simulink model "simulador2017bVALIDATION_v2"  (R2017b)
settings: Solver=FixedStepAuto  StartTime=0.0  StopTime=60*3  FixedStep=0.001  MaxStep=0.001  RelTol=1e-3
values from neighbouring files (symbols this model uses):
  b = 2.9    [FUN_v2.m]    (also in ratesDerivatives.m = (1/windowSize)*ones(1,windowSize))
  c_bar = 0.19    [FUN_v2.m]
  CD_deltae = x(5)    [FUN_v2.m]
  CDp = x(1)    [FUN_v2.m]
  CDq = x(4)    [FUN_v2.m]
  CL0 = x(6)    [FUN_v2.m]
  CL_alpha = x(7)    [FUN_v2.m]
  Cl_beta = x(15)    [FUN_v2.m]
  Cl_da = x(19)    [FUN_v2.m]
  CL_deltae = x(9)    [FUN_v2.m]
  Cl_dr = x(18)    [FUN_v2.m]
  Cl_p = x(16)    [FUN_v2.m]
  Cl_r = x(17)    [FUN_v2.m]
  CLq = x(8)    [FUN_v2.m]
  Cm0 = x(20)    [FUN_v2.m]
  Cm_alpha = x(21)    [FUN_v2.m]
  Cm_de = x(23)    [FUN_v2.m]
  Cm_q = x(22)    [FUN_v2.m]
  Cn_beta = x(24)    [FUN_v2.m]
  Cn_da = x(28)    [FUN_v2.m]
  Cn_dr = x(27)    [FUN_v2.m]
  Cn_p = x(25)    [FUN_v2.m]
  Cn_r = x(26)    [FUN_v2.m]
  Cy_beta = x(10)    [FUN_v2.m]
  Cy_da = x(13)    [FUN_v2.m]
  Cy_dr = x(14)    [FUN_v2.m]
  Cy_p = x(11)    [FUN_v2.m]
  Cy_r = x(12)    [FUN_v2.m]
  deltat_pts = parameters.deltat_pts    [propulsiveModel.m]
  k1 = x(3)    [FUN_v2.m]
  k2 = x(2)    [FUN_v2.m]
  M = parameters.M    [propulsiveModel.m]
  mass = 11    [FUN_v2.m]
  q = XDATA(:,5)    [FUN_v2.m]    (also in NONLINEAR_IDENTIFICATION_v2.m = myResize(q_meas); ratesDerivatives.m = q_meas)
  r = XDATA(:,6)    [FUN_v2.m]    (also in NONLINEAR_IDENTIFICATION_v2.m = myResize(r_meas); ratesDerivatives.m = r_meas)
  RPM_pts = parameters.RPM_pts    [propulsiveModel.m]
  T = table(xfit,xreal,relErrorPorcentage','RowNames',coeffName)    [NONLINEAR_IDENTIFICATION_v2.m]    (also in propulsiveModel.m = parameters.T)
  V = sqrt(u.*u+v.*v+w.*w)    [NoisySignals_plot.m]
undefined symbols (not defined in the file or in its folder): Cl0, Cm_df, Cn0, Cx_df, Cx_dr, Cy0, Cz_df, delta_max, Earth, F, Light, maxRPM, MIL, N, Vw_unif, WGS84
libraries: aerolibwind2 x3, aerolibtransform2 x2, aerolibasang x2, aerolibfltsims x1, simulink_extras x1, aerolibatmos2 x1, shared6dof x1, aerolibadyn x1
(part 2 of 2)

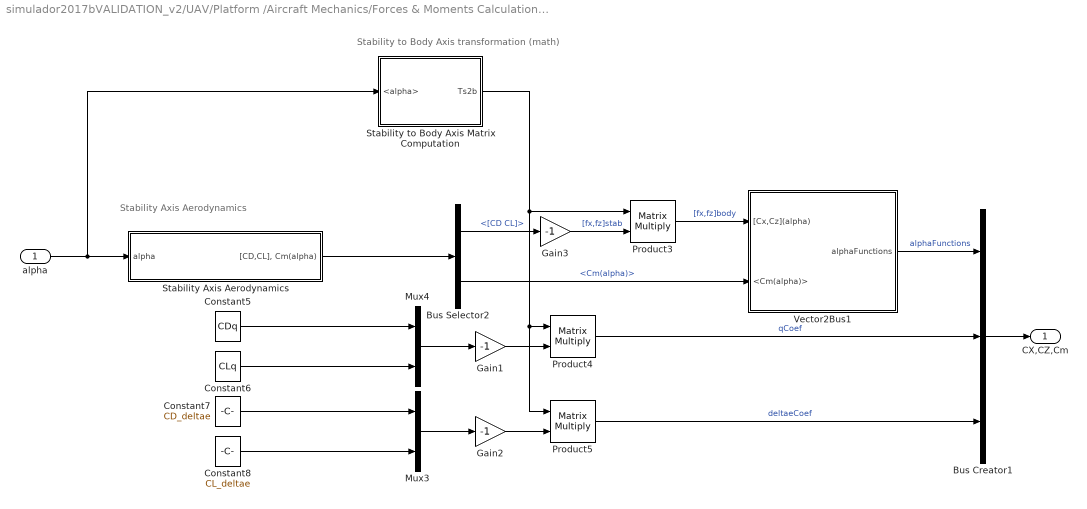
== system simulador2017bVALIDATION_v2/UAV/Platform /Aircraft Mechanics/Forces & Moments Calculation/Aerodynamic Coefficients /Longitudinal Aerodynamics (Cx, Cz, Cm coefficients) ==
  note: Stability Axis Aerodynamics
  note: Stability to Body Axis transformation (math)
  "alpha " : Inport
  Bus Creator1 : BusCreator  Inputs=3
  Bus Selector2 : BusSelector  OutputSignals=[CD CL],Cm(alpha)
  Constant5 : Constant  Value=CDq
      mask Display: port_label('output',1,'C_{D_q}','texmode','on')
  Constant6 : Constant  Value=CLq
      mask Display: port_label('output',1,'C_{L_q}','texmode','on')
  Constant7 : Constant  Value=CD_deltae
      mask Display: port_label('output',1,'C_{D_{\delta_e}}','texmode','on')
  Constant8 : Constant  Value=CL_deltae
      mask Display: port_label('output',1,'C_{L_{\delta_e}}','texmode','on')
  Gain1 : Gain  Gain=-1
  Gain2 : Gain  Gain=-1
  Gain3 : Gain  Gain=-1
  Mux3 : Mux  Inputs=2
  Mux4 : Mux  Inputs=2
  Product3 : Product  Multiplication=Matrix(*)
  Product4 : Product  Multiplication=Matrix(*)
  Product5 : Product  Multiplication=Matrix(*)
  Stability Axis Aerodynamics : Subsystem
      mask Display:
      | port_label('input',1,'\alpha','texmode','on')
      | port_label('output',1,'[C_D(\alpha),C_L(\alpha)], C_m(\alpha)','texmode','on')
  Stability to Body Axis Matrix Computation : Subsystem
      mask Display:
      | port_label('input',1,'\alpha','texmode','on')
      | port_label('output',1,'T_{s2b}(\alpha)','texmode','on')
  Vector2Bus1 : Subsystem
      mask Display:
      | port_label('input',1,'[C_X(\alpha), C_Z(\alpha)]','texmode','on')
      | port_label('input',2,'C_m(\alpha)','texmode','on')
      | port_label('output',1,'C_X(\alpha),C_Z(\alpha),C_m(\alpha)','texmode','on')
  CX,CZ,Cm : Outport
  wires:
  Bus Creator1/1 -> CX,CZ,Cm/1
  Gain3/1 -> Product3/2  "[fx,fz]stab"
  Stability Axis Aerodynamics/1("[CD,CL], Cm(alpha)") -> Bus Selector2/1
  Constant7/1 -> Mux3/1
  Stability to Body Axis Matrix Computation/1(Ts2b) -> Product5/1, Product4/1, Product3/1
  Product4/1 -> Bus Creator1/2  "qCoef"
  Bus Selector2/1 -> Gain3/1  "<[CD CL]>"
  Product5/1 -> Bus Creator1/3  "deltaeCoef"
  Product3/1 -> Vector2Bus1/1("[Cx,Cz](alpha)")  "[fx,fz]body"
  Bus Selector2/2 -> Vector2Bus1/2(<Cm(alpha)>)  "<Cm(alpha)>"
  Constant8/1 -> Mux3/2
  Vector2Bus1/1(alphaFunctions) -> Bus Creator1/1  "alphaFunctions"
  Constant6/1 -> Mux4/2
  Constant5/1 -> Mux4/1
  Mux3/1 -> Gain2/1
  Gain2/1 -> Product5/2
  Mux4/1 -> Gain1/1
  Gain1/1 -> Product4/2
  "alpha "/1 -> Stability Axis Aerodynamics/1(alpha), Stability to Body Axis Matrix Computation/1(<alpha>)

== system simulador2017bVALIDATION_v2/UAV/Platform /Aircraft Mechanics/Forces & Moments Calculation/Aerodynamic Coefficients /alpha-beta Coefficients ==
  beta : Inport  Unit=radian
  Bus Element In : Inport  Port=2  PortName=Longitudinal Aerodynamics  Element=Cm(alpha)
  Bus Element In1 : Inport  Port=2  PortName=Longitudinal Aerodynamics  Element=Cz(alpha)
  Bus Element In2 : Inport  Port=2  PortName=Longitudinal Aerodynamics  Element=Cx(alpha)
  Gain1 : Gain  Gain=Cn_beta  SaturateOnIntegerOverflow=on  OutDataTypeStr=Inherit: Same as input  ParamDataTypeStr=Inherit: Same as input
  Gain3 : Gain  Gain=Cy_beta  SaturateOnIntegerOverflow=on  OutDataTypeStr=Inherit: Same as input  ParamDataTypeStr=Inherit: Same as input
  Gain6 : Gain  Gain=Cl_beta  SaturateOnIntegerOverflow=on  OutDataTypeStr=Inherit: Same as input  ParamDataTypeStr=Inherit: Same as input
  Lateral Dynamics Constants : Constant  Value=[0,Cy0,0,Cl0,0,Cn0]
  Mux1 : Mux  Inputs=6
  Sum4 : Sum  Inputs=|++  SaturateOnIntegerOverflow=on
  Coefficients : Outport
  wires:
  Lateral Dynamics Constants/1 -> Sum4/2
  Sum4/1 -> Coefficients/1
  Mux1/1 -> Sum4/1
  Gain3/1 -> Mux1/2  "Cy"
  Gain6/1 -> Mux1/4  "Cl"
  beta/1 -> Gain1/1, Gain6/1, Gain3/1  "beta"
  Gain1/1 -> Mux1/6
  Bus Element In/1 -> Mux1/5
  Bus Element In1/1 -> Mux1/3
  Bus Element In2/1 -> Mux1/1

== system simulador2017bVALIDATION_v2/UAV/Platform /Aircraft Mechanics/Forces & Moments Calculation/Propulsion/1 dim to 6 dim1 ==
  Tprop : Inport
  Qprop : Inport  Port=2
  Bus Creator : BusCreator  Inputs=2
  Constant : Constant  Value=0
  Mux : Mux  Inputs=3
  Mux1 : Mux  Inputs=3
  Propulsion BUS : Outport
  wires:
  Bus Creator/1 -> Propulsion BUS/1
  Constant/1 -> Mux/3, Mux/2, Mux1/2, Mux1/3
  Qprop/1 -> Mux1/1
  Tprop/1 -> Mux/1
  Mux/1 -> Bus Creator/1  "Tprop"
  Mux1/1 -> Bus Creator/2  "Mprop"

== system simulador2017bVALIDATION_v2/UAV/Platform /Aircraft Mechanics/Forces & Moments Calculation/Propulsion/Propeller ==
  RPM : Inport
  u : Inport  Port=2
  1-D Lookup Table : Lookup_n-D  BreakpointsForDimension1=N  BreakpointsForDimension2=V  Table=T  InternalRulePriority=Speed  RndMeth=Simplest  InputSameDT=on
  1-D Lookup Table1 : Lookup_n-D  BreakpointsForDimension1=N  BreakpointsForDimension2=V  Table=M  InternalRulePriority=Speed  RndMeth=Simplest  InputSameDT=on
  Tables work with RPM/1000 : Gain  Gain=1/1000
  Tprop : Outport
  Qprop : Outport  Port=2
  wires:
  1-D Lookup Table/1 -> Tprop/1
  u/1 -> 1-D Lookup Table/2, 1-D Lookup Table1/2
  1-D Lookup Table1/1 -> Qprop/1
  RPM/1 -> Tables work with RPM/1000/1
  Tables work with RPM/1000/1 -> 1-D Lookup Table1/1, 1-D Lookup Table/1

== system simulador2017bVALIDATION_v2/UAV/Platform /Aircraft Mechanics/Forces & Moments Calculation/Aerodynamic Coefficients /Actuator Increments/Aileron ==
  note: Se ha despreciado el efecto del angulo de ataque,
      | que afecta a las superficies de control si es muy alto
  deltaa : Inport  Unit=rad
  Gain1 : Gain  Gain=0  SaturateOnIntegerOverflow=on  OutDataTypeStr=Inherit: Same as input  ParamDataTypeStr=Inherit: Same as input
  Gain2 : Gain  Gain=Cy_da  SaturateOnIntegerOverflow=on  OutDataTypeStr=Inherit: Same as input  ParamDataTypeStr=Inherit: Same as input
  Gain3 : Gain  Gain=0  SaturateOnIntegerOverflow=on  OutDataTypeStr=Inherit: Same as input  ParamDataTypeStr=Inherit: Same as input
  Gain4 : Gain  Gain=Cn_da  SaturateOnIntegerOverflow=on  OutDataTypeStr=Inherit: Same as input  ParamDataTypeStr=Inherit: Same as input
  Gain5 : Gain  Gain=0  SaturateOnIntegerOverflow=on  OutDataTypeStr=Inherit: Same as input  ParamDataTypeStr=Inherit: Same as input
  Gain6 : Gain  Gain=Cl_da  SaturateOnIntegerOverflow=on  OutDataTypeStr=Inherit: Same as input  ParamDataTypeStr=Inherit: Same as input
  Mux1 : Mux  Inputs=6
  delCoeff : Outport
  wires:
  Gain6/1 -> Mux1/4
  Gain1/1 -> Mux1/1  "Cx"
  Mux1/1 -> delCoeff/1
  Gain2/1 -> Mux1/2  "Cy"
  Gain3/1 -> Mux1/3  "Cz"
  Gain5/1 -> Mux1/5  "Cm"
  Gain4/1 -> Mux1/6
  deltaa/1 -> Gain2/1, Gain3/1, Gain5/1, Gain4/1, Gain6/1, Gain1/1

== system simulador2017bVALIDATION_v2/UAV/Platform /Aircraft Mechanics/Forces & Moments Calculation/Aerodynamic Coefficients /Actuator Increments/Elevator ==
  "Cx_deltae, Cz_deltae" : Inport
  deltae : Inport  Port=2
  Constant1 : Constant  Value=0
  Demux : Demux  Outputs=2
  Gain3 : Gain  Gain=Cm_de  SaturateOnIntegerOverflow=on  OutDataTypeStr=Inherit: Same as input  ParamDataTypeStr=Inherit: Same as input
  Mux1 : Mux  Inputs=6
  Product : Product
  Product1 : Product
  delCoeff : Outport
  wires:
  Gain3/1 -> Mux1/5
  Product1/1 -> Mux1/3
  Mux1/1 -> delCoeff/1
  Constant1/1 -> Mux1/4, Mux1/6, Mux1/2
  Product/1 -> Mux1/1
  "Cx_deltae, Cz_deltae"/1 -> Demux/1
  Demux/1 -> Product/1  "Cx_deltae"
  Demux/2 -> Product1/1  "Cz_deltae"
  deltae/1 -> Product/2, Product1/2, Gain3/1

== system simulador2017bVALIDATION_v2/UAV/Platform /Aircraft Mechanics/Forces & Moments Calculation/Aerodynamic Coefficients /Actuator Increments/Flap ==
  deltaf : Inport  Unit=rad
  Constant1 : Constant  Value=0
  Gain1 : Gain  Gain=Cx_df  SaturateOnIntegerOverflow=on  OutDataTypeStr=Inherit: Same as input  ParamDataTypeStr=Inherit: Same as input
  Gain3 : Gain  Gain=Cz_df  SaturateOnIntegerOverflow=on  OutDataTypeStr=Inherit: Same as input  ParamDataTypeStr=Inherit: Same as input
  Gain5 : Gain  Gain=Cm_df  SaturateOnIntegerOverflow=on  OutDataTypeStr=Inherit: Same as input  ParamDataTypeStr=Inherit: Same as input
  Mux1 : Mux  Inputs=6
  delCoeff : Outport
  wires:
  deltaf/1 -> Gain1/1, Gain3/1, Gain5/1  "df"
  Gain5/1 -> Mux1/5
  Mux1/1 -> delCoeff/1
  Constant1/1 -> Mux1/4, Mux1/6, Mux1/2
  Gain1/1 -> Mux1/1
  Gain3/1 -> Mux1/3

== system simulador2017bVALIDATION_v2/UAV/Platform /Aircraft Mechanics/Forces & Moments Calculation/Aerodynamic Coefficients /Actuator Increments/Rudder ==
  note: Se añade la contribucion en
      | resistencia del Rudder direccion X
  note: Se ha despreciado el efecto del angulo de ataque,
      | que afecta a las superficies de control si es muy alto
  deltar : Inport  Unit=rad
  Constant1 : Constant  Value=0
  Gain1 : Gain  Gain=Cl_dr  SaturateOnIntegerOverflow=on  OutDataTypeStr=Inherit: Same as input  ParamDataTypeStr=Inherit: Same as input
  Gain2 : Gain  Gain=Cn_dr  SaturateOnIntegerOverflow=on  OutDataTypeStr=Inherit: Same as input  ParamDataTypeStr=Inherit: Same as input
  Gain4 : Gain  Gain=Cy_dr  SaturateOnIntegerOverflow=on  OutDataTypeStr=Inherit: Same as input  ParamDataTypeStr=Inherit: Same as input
  Gain5 : Gain  Commented=on  Gain=Cx_dr  SaturateOnIntegerOverflow=on  OutDataTypeStr=Inherit: Same as input  ParamDataTypeStr=Inherit: Same as input
  Mux1 : Mux  Inputs=6
  delCoeff : Outport
  wires:
  Gain1/1 -> Mux1/4
  Gain2/1 -> Mux1/6
  Mux1/1 -> delCoeff/1
  Gain4/1 -> Mux1/2
  Constant1/1 -> Mux1/1, Mux1/5, Mux1/3
  deltar/1 -> Gain5/1, Gain4/1, Gain1/1, Gain2/1  "dr"

== system simulador2017bVALIDATION_v2/UAV/Platform /Aircraft Mechanics/Forces & Moments Calculation/Aerodynamic Coefficients /Body Rate Damping/p Coefficients ==
  Constant1 : Constant  Value=0
  Constant2 : Constant  Value=Cy_p
  Constant3 : Constant  Value=Cl_p
  Constant4 : Constant  Value=Cn_p
  Mux1 : Mux  Inputs=6
  p Coeff : Outport
  wires:
  Constant2/1 -> Mux1/2
  Mux1/1 -> p Coeff/1
  Constant1/1 -> Mux1/5, Mux1/3, Mux1/1
  Constant4/1 -> Mux1/6
  Constant3/1 -> Mux1/4

== system simulador2017bVALIDATION_v2/UAV/Platform /Aircraft Mechanics/Forces & Moments Calculation/Aerodynamic Coefficients /Body Rate Damping/q Coefficients ==
  qCoef : Inport
  Constant1 : Constant  Value=0
  Constant4 : Constant  Value=Cm_q
  Demux : Demux  Outputs=2
  Mux1 : Mux  Inputs=6
  delCoeff : Outport
  wires:
  Constant1/1 -> Mux1/6, Mux1/4, Mux1/2
  Constant4/1 -> Mux1/5
  Mux1/1 -> delCoeff/1
  qCoef/1 -> Demux/1
  Demux/1 -> Mux1/1  "Cx_q"
  Demux/2 -> Mux1/3  "Cz_q"

== system simulador2017bVALIDATION_v2/UAV/Platform /Aircraft Mechanics/Forces & Moments Calculation/Aerodynamic Coefficients /Body Rate Damping/r Coefficients ==
  Constant : Constant  Value=0
  Constant1 : Constant  Value=Cy_r
  Constant2 : Constant  Value=Cl_r
  Constant4 : Constant  Value=Cn_r
  Mux1 : Mux  Inputs=6
  r Coeff : Outport
  wires:
  Constant/1 -> Mux1/5, Mux1/3, Mux1/1
  Constant1/1 -> Mux1/2
  Constant4/1 -> Mux1/6
  Constant2/1 -> Mux1/4
  Mux1/1 -> r Coeff/1

== system simulador2017bVALIDATION_v2/UAV/Platform /Aircraft Mechanics/Forces & Moments Calculation/Aerodynamic Coefficients /Longitudinal Aerodynamics (Cx, Cz, Cm coefficients)/Stability Axis Aerodynamics ==
  note: CD
  alpha : Inport
  Constant1 : Constant  Value=CL0
  Constant2 : Constant  Value=Cm0
  Constant3 : Constant  Value=CDp
  Gain1 : Gain  Gain=k1
  Gain2 : Gain  Gain=k2
  Gain4 : Gain  Gain=CL_alpha
  Gain5 : Gain  Gain=Cm_alpha
  Math Function : Math  Operator=square  SaturateOnIntegerOverflow=on
  Mux : Mux  Inputs=3
  Sum : Sum  Inputs=|++
  Sum1 : Sum  Inputs=|++
  Sum2 : Sum  Inputs=+++
  Vector2Bus : Subsystem
  "[CD,CL], Cm(alpha)" : Outport
  wires:
  Gain4/1 -> Sum/1
  Gain5/1 -> Sum1/1
  Vector2Bus/1("[CD,CL], Cm") -> "[CD,CL], Cm(alpha)"/1
  Constant1/1 -> Sum/2
  Constant2/1 -> Sum1/2
  Sum1/1 -> Mux/3  "Cm"
  Mux/1 -> Vector2Bus/1("[CD,CL,Cm]")
  Sum2/1 -> Mux/1  "CD"
  Sum/1 -> Gain2/1, Math Function/1, Mux/2  "CL"
  Constant3/1 -> Sum2/3
  alpha/1 -> Gain5/1, Gain4/1
  Gain2/1 -> Sum2/2
  Math Function/1 -> Gain1/1  "CL2"
  Gain1/1 -> Sum2/1

== system simulador2017bVALIDATION_v2/UAV/Platform /Aircraft Mechanics/Forces & Moments Calculation/Aerodynamic Coefficients /Longitudinal Aerodynamics (Cx, Cz, Cm coefficients)/Stability to Body Axis Matrix Computation ==
  note: [ ]
  note: sin cos
  note: cos -sin
  note: Column 2
  note: Column 1
  <alpha> : Inport
  Cos1 : Trigonometry  Operator=cos  OutputSignalType=real
  Cos2 : Trigonometry  OutputSignalType=real
  Gain : Gain  Gain=-1
  Matrix Concatenate : Concatenate  Mode=Multidimensional array  ConcatenateDimension=2
  Mux : Mux  Inputs=2
  Mux3 : Mux  Inputs=2
  Test Display : Display
  Ts2b : Outport
  wires:
  Gain/1 -> Mux/1
  Cos2/1 -> Mux3/2, Gain/1
  Mux3/1 -> Matrix Concatenate/1
  Mux/1 -> Matrix Concatenate/2
  Cos1/1 -> Mux3/1, Mux/2
  <alpha>/1 -> Cos2/1, Cos1/1
  Matrix Concatenate/1 -> Test Display/1, Ts2b/1  "Ts2b"

== system simulador2017bVALIDATION_v2/UAV/Platform /Aircraft Mechanics/Forces & Moments Calculation/Aerodynamic Coefficients /Longitudinal Aerodynamics (Cx, Cz, Cm coefficients)/Vector2Bus1 ==
  "[Cx,Cz](alpha)" : Inport
  <Cm(alpha)> : Inport  Port=2
  Bus Creator : BusCreator  Inputs=3
  Demux : Demux  Outputs=2
  alphaFunctions : Outport
  wires:
  "[Cx,Cz](alpha)"/1 -> Demux/1
  <Cm(alpha)>/1 -> Bus Creator/3
  Demux/2 -> Bus Creator/2  "Cz(alpha)"
  Demux/1 -> Bus Creator/1  "Cx(alpha)"
  Bus Creator/1 -> alphaFunctions/1  "alphaFunctions"

== system simulador2017bVALIDATION_v2/UAV/Platform /Aircraft Mechanics/Forces & Moments Calculation/Aerodynamic Coefficients /Longitudinal Aerodynamics (Cx, Cz, Cm coefficients)/Stability Axis Aerodynamics/Vector2Bus ==
  "[CD,CL,Cm]" : Inport
  Bus Creator : BusCreator  Inputs=2
  Demux : Demux  Outputs=3
  Mux1 : Mux  Inputs=2
  "[CD,CL], Cm" : Outport
  wires:
  Demux/3 -> Bus Creator/2  "Cm(alpha)"
  Demux/1 -> Mux1/1  "CD"
  Mux1/1 -> Bus Creator/1  "[CD CL]"
  "[CD,CL,Cm]"/1 -> Demux/1
  Bus Creator/1 -> "[CD,CL], Cm"/1
  Demux/2 -> Mux1/2  "CL"

== matlab function simulador2017bVALIDATION_v2/Scopes /Visualization BOX/Cockpit Data/MATLAB Function ==
  data: uvw input; airspeed output
function airspeed = fcn(uvw)

u = uvw(1);
v = uvw(2);
w = uvw(3);

airspeed = sqrt(u^2+v^2+w^2);
airspeed = airspeed*1.94384449; % unit convertion
